simulink model "sampleModel7126_pp_1_1"  (R2018a)
settings: Solver=VariableStepAuto  StartTime=0.0  StopTime=10.0  RelTol=1e-3
undefined symbols (not defined in the file): DiscIntNeverNeededParam
libraries: simulink x367
(part 4 of 12)

== system sampleModel7126_pp_1_1/cfblk270 ==
  cfblk1 : Inport
  Action Port : ActionPort  ActionType=else
  cfblk11 : Subsystem  TreatAsAtomicUnit=on
  cfblk12 : Delay
  cfblk13 : Delay
  cfblk3 : UnitDelay  SampleTime=-1
  cfblk4 : Subsystem  TreatAsAtomicUnit=on
  cfblk5 : simulink/Continuous/PID Controller (2DOF)  Controller=PID  TimeDomain=Discrete-time  SampleTime=-1  IntegratorMethod=Forward Euler  FilterMethod=Forward Euler  Form=Parallel  UseFilter=on  ControllerParametersSource=internal  P=1  I=1  D=0  N=100  b=1  c=1  InitialConditionSource=internal  InitialConditionForIntegrator=0  InitialConditionForFilter=0  ExternalReset=none  LimitOutput=off  UpperSaturationLimit=inf  LowerSaturationLimit=-inf  LinearizeAsGain=off  AntiWindupMode=none  Kb=1  TrackingMode=off  Kt=1  PParamMin=[]  PParamMax=[]  IParamMin=[]  IParamMax=[]  DParamMin=[]  DParamMax=[]  NParamMin=[]  NParamMax=[]  bParamMin=[]  bParamMax=[]  cParamMin=[]  cParamMax=[]  KbParamMin=[]  KbParamMax=[]  KtParamMin=[]  KtParamMax=[]  POutMin=[]  POutMax=[]  IOutMin=[]  IOutMax=[]  DOutMin=[]  DOutMax=[]  NOutMin=[]  NOutMax=[]  bOutMin=[]  bOutMax=[]  cOutMin=[]  cOutMax=[]  KbOutMin=[]  KbOutMax=[]  KtOutMin=[]  KtOutMax=[]  IntegratorOutMin=[]  IntegratorOutMax=[]  FilterOutMin=[]  FilterOutMax=[]  SumOutMin=[]  SumOutMax=[]  Sum1OutMin=[]  Sum1OutMax=[]  Sum2OutMin=[]  Sum2OutMax=[]  Sum3OutMin=[]  Sum3OutMax=[]  SumI1OutMin=[]  SumI1OutMax=[]  SumI2OutMin=[]  SumI2OutMax=[]  SumI3OutMin=[]  SumI3OutMax=[]  SumDOutMin=[]  SumDOutMax=[]  SaturationOutMin=[]  SaturationOutMax=[]  IntegratorContinuousStateAttributes=''  IntegratorStateMustResolveToSignalObject=off  IntegratorRTWStateStorageClass=Auto  FilterContinuousStateAttributes=''  FilterStateMustResolveToSignalObject=off  FilterRTWStateStorageClass=Auto  DifferentiatorICPrevScaledInput=0  DifferentiatorOutMin=[]  DifferentiatorOutMax=[]  FilterDiffOutCoefMin=[]  FilterDiffOutCoefMax=[]  SumDenOutMin=[]  SumDenOutMax=[]  SumNumOutMin=[]  SumNumOutMax=[]  ReciprocalOutMin=[]  ReciprocalOutMax=[]  DivideOutMin=[]  DivideOutMax=[]  TunerSelectOption=Transfer Function Based (PID Tuner App)
  cfblk6 : simulink/Discrete/Transfer Fcn Lead or Lag  PoleZ=0.95  ZeroZ=0.75  ICPrevOutput=0.0  ICPrevInput=0.0  DoSatur=off
      settings: SourceProductName=Simulink  SourceProductBaseCode=SL
  cfblk7 : simulink/Continuous/PID Controller  Controller=PID  TimeDomain=Discrete-time  SampleTime=-1  IntegratorMethod=Forward Euler  FilterMethod=Forward Euler  Form=Parallel  UseFilter=on  ControllerParametersSource=internal  P=1  I=1  D=0  N=100  InitialConditionSource=internal  InitialConditionForIntegrator=0  InitialConditionForFilter=0  ExternalReset=none  LimitOutput=off  UpperSaturationLimit=inf  LowerSaturationLimit=-inf  LinearizeAsGain=off  AntiWindupMode=none  Kb=1  TrackingMode=off  Kt=1  PParamMin=[]  PParamMax=[]  IParamMin=[]  IParamMax=[]  DParamMin=[]  DParamMax=[]  NParamMin=[]  NParamMax=[]  KbParamMin=[]  KbParamMax=[]  KtParamMin=[]  KtParamMax=[]  POutMin=[]  POutMax=[]  IOutMin=[]  IOutMax=[]  DOutMin=[]  DOutMax=[]  NOutMin=[]  NOutMax=[]  KbOutMin=[]  KbOutMax=[]  KtOutMin=[]  KtOutMax=[]  IntegratorOutMin=[]  IntegratorOutMax=[]  FilterOutMin=[]  FilterOutMax=[]  SumOutMin=[]  SumOutMax=[]  SumI1OutMin=[]  SumI1OutMax=[]  SumI2OutMin=[]  SumI2OutMax=[]  SumI3OutMin=[]  SumI3OutMax=[]  SumDOutMin=[]  SumDOutMax=[]  SaturationOutMin=[]  SaturationOutMax=[]  IntegratorContinuousStateAttributes=''  IntegratorStateMustResolveToSignalObject=off  IntegratorRTWStateStorageClass=Auto  FilterContinuousStateAttributes=''  FilterStateMustResolveToSignalObject=off  FilterRTWStateStorageClass=Auto  DifferentiatorICPrevScaledInput=0  DifferentiatorOutMin=[]  DifferentiatorOutMax=[]  FilterDiffOutCoefMin=[]  FilterDiffOutCoefMax=[]  SumDenOutMin=[]  SumDenOutMax=[]  SumNumOutMin=[]  SumNumOutMax=[]  ReciprocalOutMin=[]  ReciprocalOutMax=[]  DivideOutMin=[]  DivideOutMax=[]  TunerSelectOption=Transfer Function Based (PID Tuner App)
  cfblk8 : Delay  ShowEnablePort=on
      settings: InputPortMap=u0,e6
  cfblk9 : Subsystem  TreatAsAtomicUnit=on
  cyemi_{675..687} (13 alike) : DataTypeConversion  OutDataTypeStr=double
  emi_2047 : Subsystem  TreatAsAtomicUnit=on
  emi_2049 : If  IfExpression=0 <= u1
  emi_2050 : DataTypeConversion  OutDataTypeStr=double
  emi_211 : Subsystem  TreatAsAtomicUnit=on
  emi_213 : If  IfExpression=0 <= u1  SampleTime=[1 0]
  emi_214 : DataTypeConversion  OutDataTypeStr=double
  emi_508 : Subsystem  TreatAsAtomicUnit=on
  emi_510 : If  IfExpression=0 <= u1  SampleTime=[1 0]
  emi_511 : DataTypeConversion  OutDataTypeStr=double
  cfblk2 : Outport
  cfblk10 : Outport  Port=2
  wires:
  cfblk5/1 -> cyemi_676/1, cyemi_679/1
  cfblk1/1 -> cfblk2/1, cfblk10/1, cyemi_683/1
  cfblk3/1 -> cyemi_681/1, cyemi_687/1, emi_511/1, emi_2050/1
  cyemi_676/1 -> cfblk12/1
  cyemi_677/1 -> cfblk13/1
  cfblk6/1 -> cyemi_677/1
  cyemi_678/1 -> cfblk3/1
  cfblk8/1 -> cyemi_678/1
  cyemi_680/1 -> cfblk5/1
  cyemi_681/1 -> cfblk5/2
  cyemi_682/1 -> cfblk6/1
  cyemi_683/1 -> cfblk7/1
  cyemi_684/1 -> cfblk8/1
  cfblk7/1 -> cyemi_684/1
  cyemi_685/1 -> cfblk8/2
  cfblk12/1 -> cyemi_685/1
  cfblk13/1 -> cyemi_686/1
  cyemi_679/1 -> cfblk4/1(emi_209)
  cfblk4/1(emi_210) -> cyemi_675/1
  emi_213/1 -> cfblk4/Action
  emi_213/2 -> emi_211/Action
  emi_214/1 -> emi_213/1
  cyemi_686/1 -> cfblk9/1(emi_505)
  cyemi_687/1 -> cfblk9/2(emi_506)
  cfblk9/1(emi_507) -> cyemi_682/1
  emi_510/1 -> cfblk9/Action
  emi_510/2 -> emi_508/Action
  emi_511/1 -> emi_510/1
  cyemi_675/1 -> cfblk11/1(emi_2045)
  cfblk11/1(emi_2046) -> emi_214/1, cyemi_680/1
  emi_2049/1 -> cfblk11/Action
  emi_2049/2 -> emi_2047/Action
  emi_2050/1 -> emi_2049/1

== system sampleModel7126_pp_1_1/cfblk271 ==
  cfblk1 : Inport
  cfblk14 : Inport  Port=2
  Action Port : ActionPort  ActionType=then
  cfblk10 : Subsystem  TreatAsAtomicUnit=on
  cfblk11 : simulink/Discrete/Difference  ICPrevInput=0.0  OutMin=[]  OutMax=[]  OutDataTypeStr=double  OutputDataTypeScalingMode=double  OutDataType=fixdt(1, 16)  OutScaling=2^-10  DoSatur=off
  cfblk12 : DiscreteZeroPole  Poles=[0 0.5]  Gain=1  SampleTime=-1
  cfblk13 : simulink/Continuous/PID Controller  Controller=PID  TimeDomain=Discrete-time  SampleTime=-1  IntegratorMethod=Forward Euler  FilterMethod=Forward Euler  Form=Parallel  UseFilter=on  ControllerParametersSource=internal  P=1  I=1  D=0  N=100  InitialConditionSource=internal  InitialConditionForIntegrator=0  InitialConditionForFilter=0  ExternalReset=none  LimitOutput=off  UpperSaturationLimit=inf  LowerSaturationLimit=-inf  LinearizeAsGain=off  AntiWindupMode=none  Kb=1  TrackingMode=off  Kt=1  PParamMin=[]  PParamMax=[]  IParamMin=[]  IParamMax=[]  DParamMin=[]  DParamMax=[]  NParamMin=[]  NParamMax=[]  KbParamMin=[]  KbParamMax=[]  KtParamMin=[]  KtParamMax=[]  POutMin=[]  POutMax=[]  IOutMin=[]  IOutMax=[]  DOutMin=[]  DOutMax=[]  NOutMin=[]  NOutMax=[]  KbOutMin=[]  KbOutMax=[]  KtOutMin=[]  KtOutMax=[]  IntegratorOutMin=[]  IntegratorOutMax=[]  FilterOutMin=[]  FilterOutMax=[]  SumOutMin=[]  SumOutMax=[]  SumI1OutMin=[]  SumI1OutMax=[]  SumI2OutMin=[]  SumI2OutMax=[]  SumI3OutMin=[]  SumI3OutMax=[]  SumDOutMin=[]  SumDOutMax=[]  SaturationOutMin=[]  SaturationOutMax=[]  IntegratorContinuousStateAttributes=''  IntegratorStateMustResolveToSignalObject=off  IntegratorRTWStateStorageClass=Auto  FilterContinuousStateAttributes=''  FilterStateMustResolveToSignalObject=off  FilterRTWStateStorageClass=Auto  DifferentiatorICPrevScaledInput=0  DifferentiatorOutMin=[]  DifferentiatorOutMax=[]  FilterDiffOutCoefMin=[]  FilterDiffOutCoefMax=[]  SumDenOutMin=[]  SumDenOutMax=[]  SumNumOutMin=[]  SumNumOutMax=[]  ReciprocalOutMin=[]  ReciprocalOutMax=[]  DivideOutMin=[]  DivideOutMax=[]  TunerSelectOption=Transfer Function Based (PID Tuner App)
  cfblk15 : Delay
  cfblk16 : Subsystem  TreatAsAtomicUnit=on
  cfblk3 : Subsystem  TreatAsAtomicUnit=on
  cfblk4 : Delay  DelayLengthSource=Input port
      settings: InputPortMap=u0,p1
  cfblk5 : simulink/Discrete/Difference  ICPrevInput=0.0  OutMin=[]  OutMax=[]  OutDataTypeStr=double  OutputDataTypeScalingMode=double  OutDataType=fixdt(1, 16)  OutScaling=2^-10  DoSatur=off
  cfblk6 : Delay  DelayLengthSource=Input port
      settings: InputPortMap=u0,p1
  cfblk7 : simulink/Continuous/PID Controller (2DOF)  Controller=PID  TimeDomain=Discrete-time  SampleTime=-1  IntegratorMethod=Forward Euler  FilterMethod=Forward Euler  Form=Parallel  UseFilter=on  ControllerParametersSource=internal  P=1  I=1  D=0  N=100  b=1  c=1  InitialConditionSource=internal  InitialConditionForIntegrator=0  InitialConditionForFilter=0  ExternalReset=none  LimitOutput=off  UpperSaturationLimit=inf  LowerSaturationLimit=-inf  LinearizeAsGain=off  AntiWindupMode=none  Kb=1  TrackingMode=off  Kt=1  PParamMin=[]  PParamMax=[]  IParamMin=[]  IParamMax=[]  DParamMin=[]  DParamMax=[]  NParamMin=[]  NParamMax=[]  bParamMin=[]  bParamMax=[]  cParamMin=[]  cParamMax=[]  KbParamMin=[]  KbParamMax=[]  KtParamMin=[]  KtParamMax=[]  POutMin=[]  POutMax=[]  IOutMin=[]  IOutMax=[]  DOutMin=[]  DOutMax=[]  NOutMin=[]  NOutMax=[]  bOutMin=[]  bOutMax=[]  cOutMin=[]  cOutMax=[]  KbOutMin=[]  KbOutMax=[]  KtOutMin=[]  KtOutMax=[]  IntegratorOutMin=[]  IntegratorOutMax=[]  FilterOutMin=[]  FilterOutMax=[]  SumOutMin=[]  SumOutMax=[]  Sum1OutMin=[]  Sum1OutMax=[]  Sum2OutMin=[]  Sum2OutMax=[]  Sum3OutMin=[]  Sum3OutMax=[]  SumI1OutMin=[]  SumI1OutMax=[]  SumI2OutMin=[]  SumI2OutMax=[]  SumI3OutMin=[]  SumI3OutMax=[]  SumDOutMin=[]  SumDOutMax=[]  SaturationOutMin=[]  SaturationOutMax=[]  IntegratorContinuousStateAttributes=''  IntegratorStateMustResolveToSignalObject=off  IntegratorRTWStateStorageClass=Auto  FilterContinuousStateAttributes=''  FilterStateMustResolveToSignalObject=off  FilterRTWStateStorageClass=Auto  DifferentiatorICPrevScaledInput=0  DifferentiatorOutMin=[]  DifferentiatorOutMax=[]  FilterDiffOutCoefMin=[]  FilterDiffOutCoefMax=[]  SumDenOutMin=[]  SumDenOutMax=[]  SumNumOutMin=[]  SumNumOutMax=[]  ReciprocalOutMin=[]  ReciprocalOutMax=[]  DivideOutMin=[]  DivideOutMax=[]  TunerSelectOption=Transfer Function Based (PID Tuner App)
  cfblk8 : UnitDelay  SampleTime=-1
  cfblk9 : simulink/Discrete/Transfer Fcn Real Zero  ZeroZ=0.75  ICPrevInput=0.0  DoSatur=off
      settings: SourceProductName=Simulink  SourceProductBaseCode=SL
  cyemi_{690..705} (16 alike) : DataTypeConversion  OutDataTypeStr=double
  emi_133 : Subsystem  TreatAsAtomicUnit=on
  emi_135 : If  IfExpression=Inf <= u1  SampleTime=[1 0]
  emi_136 : DataTypeConversion  OutDataTypeStr=double
  emi_1887 : Subsystem  TreatAsAtomicUnit=on
  emi_1889 : If  IfExpression=Inf <= u1
  emi_1890 : DataTypeConversion  OutDataTypeStr=double
  emi_1915 : Subsystem  TreatAsAtomicUnit=on
  emi_1917 : If  IfExpression=Inf <= u1  SampleTime=[1 0]
  emi_1918 : DataTypeConversion  OutDataTypeStr=double
  cfblk2 : Outport
  wires:
  cfblk13/1 -> cfblk2/1
  cfblk9/1 -> cyemi_690/1, cyemi_695/1
  cyemi_691/1 -> cfblk11/1
  cfblk14/1 -> cyemi_691/1
  cyemi_692/1 -> cfblk12/1
  cfblk1/1 -> cyemi_692/1
  cyemi_693/1 -> cfblk13/1
  cyemi_694/1 -> cfblk15/1
  cfblk5/1 -> cyemi_694/1
  cfblk6/1 -> cyemi_696/1
  cyemi_697/1 -> cfblk4/1
  cfblk8/1 -> cyemi_697/1
  cyemi_698/1 -> cfblk4/2
  cyemi_699/1 -> cfblk5/1
  cyemi_700/1 -> cfblk6/1
  cfblk15/1 -> cyemi_700/1, emi_1918/1
  cyemi_701/1 -> cfblk6/2
  cfblk12/1 -> cyemi_701/1, emi_136/1
  cyemi_702/1 -> cfblk7/1
  cfblk11/1 -> cyemi_702/1
  cyemi_703/1 -> cfblk7/2
  cyemi_704/1 -> cfblk8/1
  cfblk7/1 -> cyemi_704/1
  cyemi_705/1 -> cfblk9/1
  cfblk4/1 -> cyemi_705/1, emi_1890/1
  cyemi_695/1 -> cfblk16/1(emi_131)
  cfblk16/1(emi_132) -> cyemi_698/1
  emi_135/1 -> cfblk16/Action
  emi_135/2 -> emi_133/Action
  emi_136/1 -> emi_135/1
  cyemi_690/1 -> cfblk10/1(emi_1885)
  cfblk10/1(emi_1886) -> cyemi_699/1
  emi_1889/1 -> cfblk10/Action
  emi_1889/2 -> emi_1887/Action
  emi_1890/1 -> emi_1889/1
  cyemi_696/1 -> cfblk3/1(emi_1913)
  cfblk3/1(emi_1914) -> cyemi_703/1, cyemi_693/1
  emi_1917/1 -> cfblk3/Action
  emi_1917/2 -> emi_1915/Action
  emi_1918/1 -> emi_1917/1

== system sampleModel7126_pp_1_1/cfblk272 ==
  cfblk1 : Inport
  cfblk9 : Inport  Port=2
  Action Port : ActionPort  ActionType=else
  cfblk11 : Delay
  cfblk12 : Subsystem  TreatAsAtomicUnit=on
  cfblk13 : DataTypeConversion  OutDataTypeStr=double
  cfblk3 : Delay  ShowEnablePort=on
      settings: InputPortMap=u0,e6
  cfblk4 : Subsystem  TreatAsAtomicUnit=on
  cfblk5 : Subsystem  TreatAsAtomicUnit=on
  cfblk6 : Subsystem  TreatAsAtomicUnit=on
  cfblk7 : Subsystem  TreatAsAtomicUnit=on
  cfblk8 : UnitDelay  SampleTime=-1
  cyemi_{708..709,711..718} (10 alike) : DataTypeConversion  OutDataTypeStr=double
  cyemi_710 : DataTypeConversion  OutDataTypeStr=uint16
  emi_1033 : Subsystem  TreatAsAtomicUnit=on
  emi_{539,652,850,1035,1458} (5 alike) : If  IfExpression=0 <= u1  SampleTime=[1 0]
  emi_{540,653,851,1036,1459} (5 alike) : DataTypeConversion  OutDataTypeStr=double
  emi_1456 : Subsystem  TreatAsAtomicUnit=on
  emi_537 : Subsystem  TreatAsAtomicUnit=on
  emi_650 : Subsystem  TreatAsAtomicUnit=on
  emi_848 : Subsystem  TreatAsAtomicUnit=on
  cfblk2 : Outport
  cfblk10 : Outport  Port=2
  wires:
  cfblk3/1 -> cyemi_713/1, cyemi_718/1, emi_540/1, emi_1459/1
  cfblk1/1 -> cyemi_712/1, cyemi_715/1
  cyemi_708/1 -> cfblk11/1
  cyemi_710/1 -> cfblk13/1
  cfblk9/1 -> cyemi_710/1
  cyemi_711/1 -> cfblk3/1
  cfblk11/1 -> cyemi_711/1, emi_653/1
  cyemi_712/1 -> cfblk3/2
  cfblk8/1 -> cyemi_714/1
  cfblk13/1 -> cyemi_717/1, emi_1036/1
  cyemi_718/1 -> cfblk8/1
  cyemi_709/1 -> cfblk12/1(emi_535)
  cfblk12/1(emi_536) -> cyemi_716/1
  emi_539/1 -> cfblk12/Action
  emi_539/2 -> emi_537/Action
  emi_540/1 -> emi_539/1
  cyemi_714/1 -> cfblk5/1(emi_647)
  cyemi_715/1 -> cfblk5/2(emi_648)
  cfblk5/1(emi_649) -> cyemi_708/1
  emi_652/1 -> cfblk5/Action
  emi_652/2 -> emi_650/Action
  emi_653/1 -> emi_652/1
  cyemi_717/1 -> cfblk7/1(emi_846)
  cfblk7/1(emi_847) -> cyemi_709/1
  emi_850/1 -> cfblk7/Action
  emi_850/2 -> emi_848/Action
  emi_851/1 -> emi_850/1
  cyemi_713/1 -> cfblk4/1(emi_1031)
  cfblk4/1(emi_1032) -> emi_851/1, cfblk10/1
  emi_1035/1 -> cfblk4/Action
  emi_1035/2 -> emi_1033/Action
  emi_1036/1 -> emi_1035/1
  cyemi_716/1 -> cfblk6/1(emi_1454)
  cfblk6/1(emi_1455) -> cfblk2/1
  emi_1458/1 -> cfblk6/Action
  emi_1458/2 -> emi_1456/Action
  emi_1459/1 -> emi_1458/1

== system sampleModel7126_pp_1_1/cfblk273 ==
  cfblk1 : Inport
  cfblk8 : Inport  Port=2
  Action Port : ActionPort  ActionType=then
  cfblk10 : Subsystem  TreatAsAtomicUnit=on
  cfblk11 : Subsystem  TreatAsAtomicUnit=on
  cfblk12 : Delay
  cfblk3 : simulink/Discrete/Tapped Delay  vinit=0.0  samptime=-1  NumDelays=1  DelayOrder=Oldest  includeCurrent=off
  cfblk4 : UnitDelay  SampleTime=-1
  cfblk5 : DiscreteZeroPole  Poles=[0 0.5]  Gain=1  SampleTime=-1
  cfblk6 : Subsystem  TreatAsAtomicUnit=on
  cfblk7 : If  SampleTime=1
  cfblk9 : Subsystem  TreatAsAtomicUnit=on
  cyemi_{721..722,733..742} (12 alike) : DataTypeConversion  OutDataTypeStr=double
  emi_1994 : Subsystem  TreatAsAtomicUnit=on
  emi_1996 : If  IfExpression=-1.330790e+00 <= u1  SampleTime=[1 0]
  emi_1997 : DataTypeConversion  OutDataTypeStr=double
  emi_883 : Subsystem  TreatAsAtomicUnit=on
  emi_885 : If  IfExpression=-1.330790e+00 <= u1
  emi_886 : DataTypeConversion  OutDataTypeStr=double
  cfblk2 : Outport
  wires:
  cfblk3/1 -> cyemi_738/1, cyemi_742/1, emi_886/1, emi_1997/1
  cfblk9/1(cfblk2) -> cfblk2/1
  cfblk7/1 -> cfblk9/Action
  cfblk7/2 -> cfblk10/Action
  cyemi_721/1 -> cfblk10/1(cfblk1)
  cfblk4/1 -> cyemi_721/1
  cyemi_722/1 -> cfblk10/2(cfblk12)
  cfblk9/2(cfblk13) -> cyemi_733/1
  cyemi_734/1 -> cfblk12/1
  cfblk5/1 -> cyemi_734/1
  cyemi_735/1 -> cfblk3/1
  cfblk1/1 -> cyemi_735/1
  cyemi_736/1 -> cfblk4/1
  cfblk8/1 -> cyemi_736/1
  cyemi_737/1 -> cfblk5/1
  cfblk10/2(cfblk13) -> cyemi_737/1
  cyemi_739/1 -> cfblk7/1
  cyemi_740/1 -> cfblk9/1(cfblk1)
  cfblk10/1(cfblk2) -> cyemi_740/1
  cyemi_741/1 -> cfblk9/2(cfblk11)
  cfblk12/1 -> cyemi_741/1
  cyemi_742/1 -> cfblk9/3(cfblk12)
  cyemi_733/1 -> cfblk11/1(emi_881)
  cfblk11/1(emi_882) -> cyemi_739/1
  emi_885/1 -> cfblk11/Action
  emi_885/2 -> emi_883/Action
  emi_886/1 -> emi_885/1
  cyemi_738/1 -> cfblk6/1(emi_1992)
  cfblk6/1(emi_1993) -> cyemi_722/1
  emi_1996/1 -> cfblk6/Action
  emi_1996/2 -> emi_1994/Action
  emi_1997/1 -> emi_1996/1

== system sampleModel7126_pp_1_1/cfblk274 ==
  cfblk1 : Inport
  Action Port : ActionPort  ActionType=else
  cfblk10 : Delay
  cfblk3 : DiscreteTransferFcn
  cfblk4 : Subsystem  TreatAsAtomicUnit=on
  cfblk5 : Subsystem  TreatAsAtomicUnit=on
  cfblk6 : Subsystem  TreatAsAtomicUnit=on
  cfblk7 : Subsystem  TreatAsAtomicUnit=on
  cfblk9 : Delay
  cyemi_{754..762} (9 alike) : DataTypeConversion  OutDataTypeStr=double
  emi_1047 : Subsystem  TreatAsAtomicUnit=on
  emi_{397,893,1049,2099} (4 alike) : If  IfExpression=0 <= u1  SampleTime=[1 0]
  emi_{398,894,1050,2100} (4 alike) : DataTypeConversion  OutDataTypeStr=double
  emi_2097 : Subsystem  TreatAsAtomicUnit=on
  emi_395 : Subsystem  TreatAsAtomicUnit=on
  emi_891 : Subsystem  TreatAsAtomicUnit=on
  cfblk2 : Outport
  cfblk8 : Outport  Port=2
  wires:
  cfblk1/1 -> cfblk2/1
  cyemi_754/1 -> cfblk10/1
  cyemi_755/1 -> cfblk3/1
  cfblk10/1 -> cyemi_755/1
  cfblk9/1 -> cyemi_758/1, emi_894/1
  cfblk3/1 -> cyemi_759/1, emi_1050/1
  cyemi_762/1 -> cfblk9/1
  cyemi_756/1 -> cfblk4/1(emi_393)
  cfblk4/1(emi_394) -> cyemi_757/1
  emi_397/1 -> cfblk4/Action
  emi_397/2 -> emi_395/Action
  emi_398/1 -> emi_397/1
  cyemi_758/1 -> cfblk6/1(emi_888)
  cyemi_759/1 -> cfblk6/2(emi_889)
  cfblk6/1(emi_890) -> emi_398/1, cyemi_761/1, cyemi_760/1, emi_2100/1
  emi_893/1 -> cfblk6/Action
  emi_893/2 -> emi_891/Action
  emi_894/1 -> emi_893/1
  cyemi_757/1 -> cfblk5/1(emi_1045)
  cfblk5/1(emi_1046) -> cyemi_762/1, cyemi_754/1
  emi_1049/1 -> cfblk5/Action
  emi_1049/2 -> emi_1047/Action
  emi_1050/1 -> emi_1049/1
  cyemi_760/1 -> cfblk7/1(emi_2094)
  cyemi_761/1 -> cfblk7/2(emi_2095)
  cfblk7/1(emi_2096) -> cyemi_756/1, cfblk8/1
  emi_2099/1 -> cfblk7/Action
  emi_2099/2 -> emi_2097/Action
  emi_2100/1 -> emi_2099/1

== system sampleModel7126_pp_1_1/cfblk275 ==
  cfblk1 : Inport
  Action Port : ActionPort  ActionType=then
  cfblk10 : Subsystem  TreatAsAtomicUnit=on
  cfblk11 : Subsystem  TreatAsAtomicUnit=on
  cfblk12 : Delay
  cfblk13 : Delay
  cfblk3 : simulink/Discrete/Transfer Fcn Real Zero  ZeroZ=0.75  ICPrevInput=0.0  DoSatur=off
      settings: SourceProductName=Simulink  SourceProductBaseCode=SL
  cfblk4 : simulink/Discrete/Transfer Fcn Real Zero  ZeroZ=0.75  ICPrevInput=0.0  DoSatur=off
      settings: SourceProductName=Simulink  SourceProductBaseCode=SL
  cfblk5 : simulink/Continuous/PID Controller  Controller=PID  TimeDomain=Discrete-time  SampleTime=-1  IntegratorMethod=Forward Euler  FilterMethod=Forward Euler  Form=Parallel  UseFilter=on  ControllerParametersSource=internal  P=1  I=1  D=0  N=100  InitialConditionSource=internal  InitialConditionForIntegrator=0  InitialConditionForFilter=0  ExternalReset=none  LimitOutput=off  UpperSaturationLimit=inf  LowerSaturationLimit=-inf  LinearizeAsGain=off  AntiWindupMode=none  Kb=1  TrackingMode=off  Kt=1  PParamMin=[]  PParamMax=[]  IParamMin=[]  IParamMax=[]  DParamMin=[]  DParamMax=[]  NParamMin=[]  NParamMax=[]  KbParamMin=[]  KbParamMax=[]  KtParamMin=[]  KtParamMax=[]  POutMin=[]  POutMax=[]  IOutMin=[]  IOutMax=[]  DOutMin=[]  DOutMax=[]  NOutMin=[]  NOutMax=[]  KbOutMin=[]  KbOutMax=[]  KtOutMin=[]  KtOutMax=[]  IntegratorOutMin=[]  IntegratorOutMax=[]  FilterOutMin=[]  FilterOutMax=[]  SumOutMin=[]  SumOutMax=[]  SumI1OutMin=[]  SumI1OutMax=[]  SumI2OutMin=[]  SumI2OutMax=[]  SumI3OutMin=[]  SumI3OutMax=[]  SumDOutMin=[]  SumDOutMax=[]  SaturationOutMin=[]  SaturationOutMax=[]  IntegratorContinuousStateAttributes=''  IntegratorStateMustResolveToSignalObject=off  IntegratorRTWStateStorageClass=Auto  FilterContinuousStateAttributes=''  FilterStateMustResolveToSignalObject=off  FilterRTWStateStorageClass=Auto  DifferentiatorICPrevScaledInput=0  DifferentiatorOutMin=[]  DifferentiatorOutMax=[]  FilterDiffOutCoefMin=[]  FilterDiffOutCoefMax=[]  SumDenOutMin=[]  SumDenOutMax=[]  SumNumOutMin=[]  SumNumOutMax=[]  ReciprocalOutMin=[]  ReciprocalOutMax=[]  DivideOutMin=[]  DivideOutMax=[]  TunerSelectOption=Transfer Function Based (PID Tuner App)
  cfblk6 : simulink/Discrete/Difference  ICPrevInput=0.0  OutMin=[]  OutMax=[]  OutDataTypeStr=double  OutputDataTypeScalingMode=double  OutDataType=fixdt(1, 16)  OutScaling=2^-10  DoSatur=off
  cfblk7 : DiscreteStateSpace  SampleTime=-1
  cfblk8 : DiscreteIntegrator  SampleTime=-1  OutDataTypeStr=double  ICPrevOutput=DiscIntNeverNeededParam  ICPrevScaledInput=DiscIntNeverNeededParam
  cfblk9 : If  SampleTime=1
  cyemi_{764,777,792..800} (11 alike) : DataTypeConversion  OutDataTypeStr=double
  cfblk2 : Outport
  wires:
  cfblk1/1 -> cfblk2/1
  cfblk9/1 -> cfblk10/Action
  cfblk9/2 -> cfblk11/Action
  cyemi_764/1 -> cfblk10/1(cfblk1)
  cfblk11/2(cfblk15) -> cyemi_764/1
  cyemi_777/1 -> cfblk11/1(cfblk1)
  cfblk13/1 -> cyemi_777/1
  cyemi_792/1 -> cfblk12/1
  cfblk5/1 -> cyemi_792/1
  cyemi_793/1 -> cfblk13/1
  cfblk8/1 -> cyemi_793/1
  cyemi_794/1 -> cfblk3/1
  cfblk12/1 -> cyemi_794/1
  cyemi_795/1 -> cfblk4/1
  cfblk6/1 -> cyemi_795/1
  cyemi_796/1 -> cfblk5/1
  cfblk11/1(cfblk2) -> cyemi_796/1
  cyemi_797/1 -> cfblk6/1
  cfblk3/1 -> cyemi_797/1
  cyemi_798/1 -> cfblk7/1
  cfblk11/3(cfblk16) -> cyemi_798/1
  cyemi_799/1 -> cfblk8/1
  cfblk7/1 -> cyemi_799/1
  cyemi_800/1 -> cfblk9/1
  cfblk4/1 -> cyemi_800/1

== system sampleModel7126_pp_1_1/cfblk276 ==
  cfblk1 : Inport
  cfblk9 : Inport  Port=2
  cfblk10 : Inport  Port=3
  cfblk11 : Inport  Port=4
  Action Port : ActionPort  ActionType=else
  cfblk14 : Subsystem  TreatAsAtomicUnit=on
  cfblk3 : Subsystem  TreatAsAtomicUnit=on
  cfblk4 : Subsystem  TreatAsAtomicUnit=on
  cfblk5 : Subsystem  TreatAsAtomicUnit=on
  cfblk6 : Subsystem  TreatAsAtomicUnit=on
  cfblk7 : Subsystem  TreatAsAtomicUnit=on
  cfblk8 : Delay
  cyemi_{805..811} (7 alike) : DataTypeConversion  OutDataTypeStr=double
  cyemi_812 : DataTypeConversion  OutDataTypeStr=uint8
  emi_1105 : Subsystem  TreatAsAtomicUnit=on
  emi_{83,242,771,1107,1359} (5 alike) : If  IfExpression=0 <= u1  SampleTime=[1 0]
  emi_1108 : DataTypeConversion  OutDataTypeStr=double
  emi_1357 : Subsystem  TreatAsAtomicUnit=on
  emi_1360 : DataTypeConversion  OutDataTypeStr=uint8
  emi_1822 : Subsystem  TreatAsAtomicUnit=on
  emi_1824 : If  IfExpression=0 <= u1
  emi_1825 : DataTypeConversion  OutDataTypeStr=double
  emi_240 : Subsystem  TreatAsAtomicUnit=on
  emi_243 : DataTypeConversion  OutDataTypeStr=uint8
  emi_769 : Subsystem  TreatAsAtomicUnit=on
  emi_772 : DataTypeConversion  OutDataTypeStr=uint8
  emi_81 : Subsystem  TreatAsAtomicUnit=on
  emi_84 : DataTypeConversion  OutDataTypeStr=double
  cfblk2 : Outport
  cfblk12 : Outport  Port=2
  cfblk13 : Outport  Port=3
  wires:
  cfblk9/1 -> cfblk2/1
  cfblk11/1 -> cfblk13/1
  cfblk8/1 -> cfblk12/1, emi_243/1, emi_772/1, emi_1360/1
  cfblk10/1 -> cyemi_809/1
  cyemi_812/1 -> cfblk8/1
  cfblk1/1 -> cyemi_812/1
  cyemi_807/1 -> cfblk4/1(emi_79)
  cfblk4/1(emi_80) -> cyemi_811/1, emi_1825/1
  emi_83/1 -> cfblk4/Action
  emi_83/2 -> emi_81/Action
  emi_84/1 -> emi_83/1
  cyemi_806/1 -> cfblk3/1(emi_238)
  cfblk3/1(emi_239) -> cyemi_808/1
  emi_242/1 -> cfblk3/Action
  emi_242/2 -> emi_240/Action
  emi_243/1 -> emi_242/1
  cyemi_808/1 -> cfblk5/1(emi_767)
  cfblk5/1(emi_768) -> cyemi_807/1
  emi_771/1 -> cfblk5/Action
  emi_771/2 -> emi_769/Action
  emi_772/1 -> emi_771/1
  cyemi_809/1 -> cfblk6/1(emi_1102)
  cyemi_810/1 -> cfblk6/2(emi_1103)
  cfblk6/1(emi_1104) -> cyemi_805/1
  emi_1107/1 -> cfblk6/Action
  emi_1107/2 -> emi_1105/Action
  emi_1108/1 -> emi_1107/1
  cyemi_811/1 -> cfblk7/1(emi_1355)
  cfblk7/1(emi_1356) -> cyemi_810/1
  emi_1359/1 -> cfblk7/Action
  emi_1359/2 -> emi_1357/Action
  emi_1360/1 -> emi_1359/1
  cyemi_805/1 -> cfblk14/1(emi_1820)
  cfblk14/1(emi_1821) -> emi_1108/1, emi_84/1, cyemi_806/1
  emi_1824/1 -> cfblk14/Action
  emi_1824/2 -> emi_1822/Action
  emi_1825/1 -> emi_1824/1

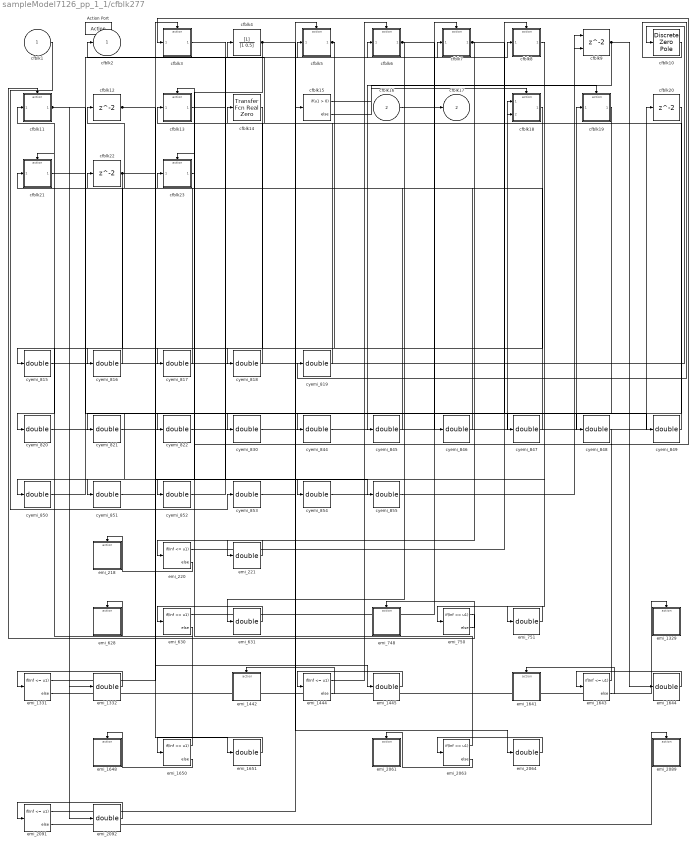
== system sampleModel7126_pp_1_1/cfblk277 ==
  cfblk1 : Inport
  cfblk16 : Inport  Port=2
  Action Port : ActionPort  ActionType=then
  cfblk10 : DiscreteZeroPole  Poles=[0 0.5]  Gain=1  SampleTime=-1
  cfblk11 : Subsystem  TreatAsAtomicUnit=on
  cfblk12 : Delay
  cfblk13 : Subsystem  TreatAsAtomicUnit=on
  cfblk14 : simulink/Discrete/Transfer Fcn Real Zero  ZeroZ=0.75  ICPrevInput=0.0  DoSatur=off
      settings: SourceProductName=Simulink  SourceProductBaseCode=SL
  cfblk15 : If  SampleTime=1
  cfblk18 : Subsystem  TreatAsAtomicUnit=on
  cfblk19 : Subsystem  TreatAsAtomicUnit=on
  cfblk20 : Delay
  cfblk21 : Subsystem  TreatAsAtomicUnit=on
  cfblk22 : Delay
  cfblk23 : Subsystem  TreatAsAtomicUnit=on
  cfblk3 : Subsystem  TreatAsAtomicUnit=on
  cfblk4 : DiscreteFilter
  cfblk5 : Subsystem  TreatAsAtomicUnit=on
  cfblk6 : Subsystem  TreatAsAtomicUnit=on
  cfblk7 : Subsystem  TreatAsAtomicUnit=on
  cfblk8 : Subsystem  TreatAsAtomicUnit=on
  cfblk9 : Delay  ShowEnablePort=on
      settings: InputPortMap=u0,e6
  cyemi_{815..822,830,844..855} (21 alike) : DataTypeConversion  OutDataTypeStr=double
  emi_1329 : Subsystem  TreatAsAtomicUnit=on
  emi_{220,630,750,1331,1643,1650,2063,2091} (8 alike) : If  IfExpression=Inf <= u1  SampleTime=[1 0]
  emi_{221,631,751,1332,1445,1644,1651,2064,2092} (9 alike) : DataTypeConversion  OutDataTypeStr=double
  emi_1442 : Subsystem  TreatAsAtomicUnit=on
  emi_1444 : If  IfExpression=Inf <= u1  SampleTime=[0 1]
  emi_1641 : Subsystem  TreatAsAtomicUnit=on
  emi_1648 : Subsystem  TreatAsAtomicUnit=on
  emi_2061 : Subsystem  TreatAsAtomicUnit=on
  emi_2089 : Subsystem  TreatAsAtomicUnit=on
  emi_218 : Subsystem  TreatAsAtomicUnit=on
  emi_628 : Subsystem  TreatAsAtomicUnit=on
  emi_748 : Subsystem  TreatAsAtomicUnit=on
  cfblk2 : Outport
  cfblk17 : Outport  Port=2
  wires:
  cfblk12/1 -> cyemi_830/1, cyemi_855/1, emi_1445/1
  cfblk16/1 -> cfblk17/1
  cfblk4/1 -> cfblk2/1, cyemi_822/1, emi_2064/1
  cfblk15/1 -> cfblk18/Action
  cfblk15/2 -> cfblk19/Action
  cyemi_815/1 -> cfblk10/1
  cfblk18/1(cfblk2) -> cyemi_816/1
  cyemi_817/1 -> cfblk12/1
  cfblk14/1 -> cyemi_818/1
  cyemi_819/1 -> cfblk14/1
  cfblk10/1 -> cyemi_819/1
  cyemi_820/1 -> cfblk15/1
  cfblk22/1 -> cyemi_820/1, emi_1651/1
  cyemi_821/1 -> cfblk18/1(cfblk1)
  cfblk20/1 -> cyemi_821/1
  cyemi_822/1 -> cfblk18/2(cfblk8)
  cyemi_830/1 -> cfblk19/1(cfblk1)
  cyemi_844/1 -> cfblk20/1
  cfblk9/1 -> cyemi_845/1, emi_751/1, emi_1644/1
  cyemi_846/1 -> cfblk22/1
  cyemi_849/1 -> cfblk4/1
  cfblk19/1(cfblk2) -> cyemi_851/1
  cfblk1/1 -> cyemi_853/1
  cyemi_854/1 -> cfblk9/1
  cyemi_855/1 -> cfblk9/2
  cyemi_853/1 -> cfblk8/1(emi_216)
  cfblk8/1(emi_217) -> cyemi_852/1
  emi_220/1 -> cfblk8/Action
  emi_220/2 -> emi_218/Action
  emi_221/1 -> emi_220/1
  cyemi_852/1 -> cfblk7/1(emi_626)
  cfblk7/1(emi_627) -> emi_221/1, cyemi_849/1
  emi_630/1 -> cfblk7/Action
  emi_630/2 -> emi_628/Action
  emi_631/1 -> emi_630/1
  cyemi_816/1 -> cfblk11/1(emi_746)
  cfblk11/1(emi_747) -> cyemi_844/1, emi_1332/1, emi_2092/1
  emi_750/1 -> cfblk11/Action
  emi_750/2 -> emi_748/Action
  emi_751/1 -> emi_750/1
  cyemi_848/1 -> cfblk3/1(emi_1327)
  cfblk3/1(emi_1328) -> cyemi_854/1
  emi_1331/1 -> cfblk3/Action
  emi_1331/2 -> emi_1329/Action
  emi_1332/1 -> emi_1331/1
  cyemi_851/1 -> cfblk6/1(emi_1440)
  cfblk6/1(emi_1441) -> emi_631/1, cyemi_846/1
  emi_1444/1 -> cfblk6/Action
  emi_1444/2 -> emi_1442/Action
  emi_1445/1 -> emi_1444/1
  cyemi_818/1 -> cfblk13/1(emi_1639)
  cfblk13/1(emi_1640) -> cyemi_847/1
  emi_1643/1 -> cfblk13/Action
  emi_1643/2 -> emi_1641/Action
  emi_1644/1 -> emi_1643/1
  cyemi_845/1 -> cfblk21/1(emi_1646)
  cfblk21/1(emi_1647) -> cyemi_848/1
  emi_1650/1 -> cfblk21/Action
  emi_1650/2 -> emi_1648/Action
  emi_1651/1 -> emi_1650/1
  cyemi_847/1 -> cfblk23/1(emi_2059)
  cfblk23/1(emi_2060) -> cyemi_850/1
  emi_2063/1 -> cfblk23/Action
  emi_2063/2 -> emi_2061/Action
  emi_2064/1 -> emi_2063/1
  cyemi_850/1 -> cfblk5/1(emi_2087)
  cfblk5/1(emi_2088) -> cyemi_817/1, cyemi_815/1
  emi_2091/1 -> cfblk5/Action
  emi_2091/2 -> emi_2089/Action
  emi_2092/1 -> emi_2091/1

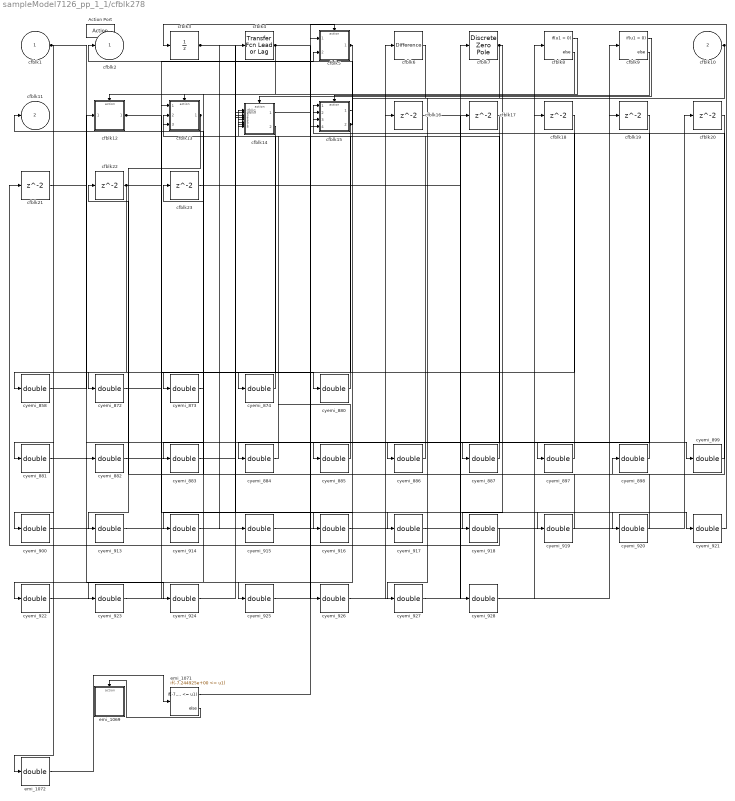
== system sampleModel7126_pp_1_1/cfblk278 ==
  cfblk1 : Inport
  cfblk10 : Inport  Port=2
  Action Port : ActionPort  ActionType=else
  cfblk12 : Subsystem  TreatAsAtomicUnit=on
  cfblk13 : Subsystem  TreatAsAtomicUnit=on
  cfblk14 : Subsystem  TreatAsAtomicUnit=on
  cfblk15 : Subsystem  TreatAsAtomicUnit=on
  cfblk{16..23} (8 alike) : Delay
  cfblk3 : UnitDelay  SampleTime=-1
  cfblk4 : simulink/Discrete/Transfer Fcn Lead or Lag  PoleZ=0.95  ZeroZ=0.75  ICPrevOutput=0.0  ICPrevInput=0.0  DoSatur=off
      settings: SourceProductName=Simulink  SourceProductBaseCode=SL
  cfblk5 : Subsystem  TreatAsAtomicUnit=on
  cfblk6 : simulink/Discrete/Difference  ICPrevInput=0.0  OutMin=[]  OutMax=[]  OutDataTypeStr=double  OutputDataTypeScalingMode=double  OutDataType=fixdt(1, 16)  OutScaling=2^-10  DoSatur=off
  cfblk7 : DiscreteZeroPole  Poles=[0 0.5]  Gain=1  SampleTime=-1
  cfblk8 : If  SampleTime=1
  cfblk9 : If  SampleTime=1
  cyemi_{858,872..874,880..887,897..900,913..928} (32 alike) : DataTypeConversion  OutDataTypeStr=double
  emi_1069 : Subsystem  TreatAsAtomicUnit=on
  emi_1071 : If  IfExpression=-7.244925e+00 <= u1  SampleTime=[1 0]
  emi_1072 : DataTypeConversion  OutDataTypeStr=double
  cfblk2 : Outport
  cfblk11 : Outport  Port=2
  wires:
  cfblk13/1(cfblk2) -> cfblk11/1, cyemi_913/1
  cfblk12/1(cfblk2) -> cyemi_917/1, cyemi_921/1
  cfblk1/1 -> cyemi_881/1, cyemi_897/1, cyemi_900/1, cyemi_924/1
  cfblk7/1 -> cyemi_918/1, cyemi_927/1
  cfblk4/1 -> cyemi_919/1, cyemi_920/1, cyemi_923/1
  cfblk3/1 -> cyemi_915/1, cyemi_916/1
  cfblk10/1 -> cyemi_886/1, cyemi_925/1
  cfblk15/2(cfblk16) -> cfblk2/1, cyemi_883/1, cyemi_885/1
  cfblk8/1 -> cfblk12/Action
  cfblk8/2 -> cfblk13/Action
  cfblk9/1 -> cfblk14/Action
  cfblk9/2 -> cfblk15/Action
  cyemi_858/1 -> cfblk12/1(cfblk1)
  cfblk14/2(cfblk16) -> cyemi_858/1
  cyemi_872/1 -> cfblk13/1(cfblk1)
  cyemi_873/1 -> cfblk13/2(cfblk8)
  cfblk6/1 -> cyemi_873/1
  cyemi_874/1 -> cfblk13/3(cfblk9)
  cfblk18/1 -> cyemi_874/1
  cyemi_880/1 -> cfblk14/1(cfblk1)
  cfblk22/1 -> cyemi_880/1, emi_1072/1
  cyemi_881/1 -> cfblk14/2(cfblk9)
  cyemi_882/1 -> cfblk14/3(cfblk10)
  cfblk21/1 -> cyemi_882/1
  cyemi_883/1 -> cfblk14/4(cfblk11)
  cyemi_884/1 -> cfblk14/5(cfblk12)
  cfblk17/1 -> cyemi_884/1
  cyemi_885/1 -> cfblk14/6(cfblk13)
  cyemi_886/1 -> cfblk14/7(cfblk14)
  cyemi_887/1 -> cfblk14/8(cfblk15)
  cfblk19/1 -> cyemi_887/1
  cyemi_897/1 -> cfblk15/1(cfblk1)
  cyemi_898/1 -> cfblk15/2(cfblk13)
  cfblk20/1 -> cyemi_898/1
  cyemi_899/1 -> cfblk15/3(cfblk14)
  cfblk16/1 -> cyemi_899/1
  cyemi_900/1 -> cfblk15/4(cfblk15)
  cyemi_913/1 -> cfblk16/1
  cyemi_914/1 -> cfblk17/1
  cyemi_915/1 -> cfblk18/1
  cyemi_916/1 -> cfblk19/1
  cyemi_917/1 -> cfblk20/1
  cyemi_918/1 -> cfblk21/1
  cyemi_919/1 -> cfblk22/1
  cyemi_920/1 -> cfblk23/1
  cyemi_921/1 -> cfblk3/1
  cyemi_922/1 -> cfblk4/1
  cfblk15/1(cfblk2) -> cyemi_922/1
  cyemi_925/1 -> cfblk6/1
  cyemi_926/1 -> cfblk7/1
  cfblk14/1(cfblk2) -> cyemi_926/1
  cyemi_927/1 -> cfblk8/1
  cyemi_928/1 -> cfblk9/1
  cfblk23/1 -> cyemi_928/1
  cyemi_923/1 -> cfblk5/1(emi_1066)
  cyemi_924/1 -> cfblk5/2(emi_1067)
  cfblk5/1(emi_1068) -> cyemi_914/1, cyemi_872/1
  emi_1071/1 -> cfblk5/Action
  emi_1071/2 -> emi_1069/Action
  emi_1072/1 -> emi_1071/1

== system sampleModel7126_pp_1_1/cfblk279 ==
  cfblk1 : Inport
  cfblk8 : Inport  Port=2
  Action Port : ActionPort  ActionType=then
  cfblk10 : Subsystem  TreatAsAtomicUnit=on
  cfblk11 : Subsystem  TreatAsAtomicUnit=on
  cfblk3 : Subsystem  TreatAsAtomicUnit=on
  cfblk4 : Subsystem  TreatAsAtomicUnit=on
  cfblk5 : DiscreteTransferFcn
  cfblk6 : DiscreteStateSpace  SampleTime=-1
  cfblk7 : Subsystem  TreatAsAtomicUnit=on
  cyemi_{931..938} (8 alike) : DataTypeConversion  OutDataTypeStr=double
  emi_1090 : Subsystem  TreatAsAtomicUnit=on
  emi_1092 : If  IfExpression=0 <= u1
  emi_{6,688,809,1093,1178} (5 alike) : DataTypeConversion  OutDataTypeStr=double
  emi_1175 : Subsystem  TreatAsAtomicUnit=on
  emi_{5,687,808,1177} (4 alike) : If  IfExpression=0 <= u1  SampleTime=[1 0]
  emi_3 : Subsystem  TreatAsAtomicUnit=on
  emi_685 : Subsystem  TreatAsAtomicUnit=on
  emi_806 : Subsystem  TreatAsAtomicUnit=on
  cfblk2 : Outport
  cfblk9 : Outport  Port=2
  wires:
  cfblk1/1 -> cfblk9/1
  cfblk5/1 -> cfblk2/1, cyemi_931/1, emi_1093/1
  cfblk6/1 -> cyemi_932/1, emi_6/1, emi_688/1
  cfblk8/1 -> cyemi_933/1
  cyemi_935/1 -> cfblk5/1
  cyemi_936/1 -> cfblk6/1
  cyemi_934/1 -> cfblk4/1(emi_1)
  cfblk4/1(emi_2) -> cyemi_936/1
  emi_5/1 -> cfblk4/Action
  emi_5/2 -> emi_3/Action
  emi_6/1 -> emi_5/1
  cyemi_932/1 -> cfblk11/1(emi_683)
  cfblk11/1(emi_684) -> cyemi_934/1, emi_809/1, emi_1178/1
  emi_687/1 -> cfblk11/Action
  emi_687/2 -> emi_685/Action
  emi_688/1 -> emi_687/1
  cyemi_937/1 -> cfblk7/1(emi_803)
  cyemi_938/1 -> cfblk7/2(emi_804)
  cfblk7/1(emi_805) -> cyemi_935/1
  emi_808/1 -> cfblk7/Action
  emi_808/2 -> emi_806/Action
  emi_809/1 -> emi_808/1
  cyemi_931/1 -> cfblk10/1(emi_1088)
  cfblk10/1(emi_1089) -> cyemi_938/1
  emi_1092/1 -> cfblk10/Action
  emi_1092/2 -> emi_1090/Action
  emi_1093/1 -> emi_1092/1
  cyemi_933/1 -> cfblk3/1(emi_1173)
  cfblk3/1(emi_1174) -> cyemi_937/1
  emi_1177/1 -> cfblk3/Action
  emi_1177/2 -> emi_1175/Action
  emi_1178/1 -> emi_1177/1

== system sampleModel7126_pp_1_1/cfblk280 ==
  cfblk1 : Inport
  cfblk10 : Inport  Port=2
  Action Port : ActionPort  ActionType=else
  cfblk13 : Subsystem  TreatAsAtomicUnit=on
  cfblk14 : Subsystem  TreatAsAtomicUnit=on
  cfblk15 : Delay
  cfblk16 : Subsystem  TreatAsAtomicUnit=on
  cfblk3 : Delay  DelayLengthSource=Input port
      settings: InputPortMap=u0,p1
  cfblk4 : Subsystem  TreatAsAtomicUnit=on
  cfblk5 : simulink/Discrete/Transfer Fcn First Order  PoleZ=0.95  ICPrevOutput=0.0  DoSatur=off
      settings: SourceProductName=Simulink
  cfblk6 : simulink/Discrete/Tapped Delay  vinit=0.0  samptime=-1  NumDelays=1  DelayOrder=Oldest  includeCurrent=off
  cfblk7 : simulink/Discrete/Transfer Fcn Lead or Lag  PoleZ=0.95  ZeroZ=0.75  ICPrevOutput=0.0  ICPrevInput=0.0  DoSatur=off
      settings: SourceProductName=Simulink  SourceProductBaseCode=SL
  cfblk8 : Delay  ShowEnablePort=on
      settings: InputPortMap=u0,e6
  cfblk9 : If  SampleTime=1
  cyemi_{942,961,963,965,969..970} (6 alike) : DataTypeConversion  OutDataTypeStr=double
  cyemi_{951,953,966..968} (5 alike) : DataTypeConversion  OutDataTypeStr=uint8
  cyemi_952 : DataTypeConversion  OutDataTypeStr=fixdt('ufix8_E6')
  cyemi_960 : DataTypeConversion  OutDataTypeStr=fixdt('ufix8_E6')
  cyemi_962 : DataTypeConversion  OutDataTypeStr=fixdt('ufix8_E3')
  cyemi_964 : DataTypeConversion  OutDataTypeStr=fixdt('ufix8_E3')
  emi_310 : Subsystem  TreatAsAtomicUnit=on
  emi_312 : If  IfExpression=Inf <= u1  SampleTime=[1 0]
  emi_313 : DataTypeConversion  OutDataTypeStr=double
  emi_360 : Subsystem  TreatAsAtomicUnit=on
  emi_362 : If  IfExpression=Inf <= u1  SampleTime=[1 0]
  emi_363 : DataTypeConversion  OutDataTypeStr=double
  cfblk2 : Outport
  cfblk11 : Outport  Port=2
  cfblk12 : Outport  Port=3
  wires:
  cfblk1/1 -> cfblk11/1, cyemi_953/1, cyemi_966/1
  cfblk10/1 -> cyemi_942/1, cyemi_969/1
  cfblk7/1 -> cfblk12/1, cyemi_962/1
  cfblk14/2(cfblk10) -> cfblk2/1
  cfblk9/1 -> cfblk13/Action
  cfblk9/2 -> cfblk14/Action
  cyemi_942/1 -> cfblk13/1(cfblk1)
  cyemi_951/1 -> cfblk14/1(cfblk1)
  cfblk6/1 -> cyemi_951/1
  cyemi_952/1 -> cfblk14/2(cfblk8)
  cfblk15/1 -> cyemi_952/1
  cyemi_953/1 -> cfblk14/3(cfblk9)
  cyemi_960/1 -> cfblk15/1
  cfblk13/2(cfblk8) -> cyemi_961/1
  cyemi_962/1 -> cfblk3/1
  cyemi_963/1 -> cfblk3/2
  cfblk5/1 -> cyemi_963/1
  cfblk3/1 -> cyemi_964/1
  cyemi_965/1 -> cfblk5/1
  cfblk13/1(cfblk2) -> cyemi_965/1
  cyemi_966/1 -> cfblk6/1
  cyemi_967/1 -> cfblk7/1
  cfblk8/1 -> cyemi_967/1, emi_313/1
  cyemi_968/1 -> cfblk8/1
  cfblk14/1(cfblk2) -> cyemi_968/1
  cyemi_969/1 -> cfblk8/2
  cyemi_970/1 -> cfblk9/1
  cyemi_961/1 -> cfblk16/1(emi_308)
  cfblk16/1(emi_309) -> cyemi_970/1, emi_363/1
  emi_312/1 -> cfblk16/Action
  emi_312/2 -> emi_310/Action
  emi_313/1 -> emi_312/1
  cyemi_964/1 -> cfblk4/1(emi_358)
  cfblk4/1(emi_359) -> cyemi_960/1
  emi_362/1 -> cfblk4/Action
  emi_362/2 -> emi_360/Action
  emi_363/1 -> emi_362/1

== system sampleModel7126_pp_1_1/cfblk281 ==
  cfblk1 : Inport
  cfblk12 : Inport  Port=2
  cfblk13 : Inport  Port=3
  Action Port : ActionPort  ActionType=then
  cfblk10 : Delay
  cfblk11 : simulink/Discrete/Transfer Fcn First Order  PoleZ=0.95  ICPrevOutput=0.0  DoSatur=off
      settings: SourceProductName=Simulink
  cfblk3 : Subsystem  TreatAsAtomicUnit=on
  cfblk4 : simulink/Continuous/PID Controller  Controller=PID  TimeDomain=Discrete-time  SampleTime=-1  IntegratorMethod=Forward Euler  FilterMethod=Forward Euler  Form=Parallel  UseFilter=on  ControllerParametersSource=internal  P=1  I=1  D=0  N=100  InitialConditionSource=internal  InitialConditionForIntegrator=0  InitialConditionForFilter=0  ExternalReset=none  LimitOutput=off  UpperSaturationLimit=inf  LowerSaturationLimit=-inf  LinearizeAsGain=off  AntiWindupMode=none  Kb=1  TrackingMode=off  Kt=1  PParamMin=[]  PParamMax=[]  IParamMin=[]  IParamMax=[]  DParamMin=[]  DParamMax=[]  NParamMin=[]  NParamMax=[]  KbParamMin=[]  KbParamMax=[]  KtParamMin=[]  KtParamMax=[]  POutMin=[]  POutMax=[]  IOutMin=[]  IOutMax=[]  DOutMin=[]  DOutMax=[]  NOutMin=[]  NOutMax=[]  KbOutMin=[]  KbOutMax=[]  KtOutMin=[]  KtOutMax=[]  IntegratorOutMin=[]  IntegratorOutMax=[]  FilterOutMin=[]  FilterOutMax=[]  SumOutMin=[]  SumOutMax=[]  SumI1OutMin=[]  SumI1OutMax=[]  SumI2OutMin=[]  SumI2OutMax=[]  SumI3OutMin=[]  SumI3OutMax=[]  SumDOutMin=[]  SumDOutMax=[]  SaturationOutMin=[]  SaturationOutMax=[]  IntegratorContinuousStateAttributes=''  IntegratorStateMustResolveToSignalObject=off  IntegratorRTWStateStorageClass=Auto  FilterContinuousStateAttributes=''  FilterStateMustResolveToSignalObject=off  FilterRTWStateStorageClass=Auto  DifferentiatorICPrevScaledInput=0  DifferentiatorOutMin=[]  DifferentiatorOutMax=[]  FilterDiffOutCoefMin=[]  FilterDiffOutCoefMax=[]  SumDenOutMin=[]  SumDenOutMax=[]  SumNumOutMin=[]  SumNumOutMax=[]  ReciprocalOutMin=[]  ReciprocalOutMax=[]  DivideOutMin=[]  DivideOutMax=[]  TunerSelectOption=Transfer Function Based (PID Tuner App)
  cfblk5 : Delay  ShowEnablePort=on
      settings: InputPortMap=u0,e6
  cfblk6 : Delay
  cfblk7 : Delay  DelayLengthSource=Input port
      settings: InputPortMap=u0,p1
  cfblk8 : DiscreteStateSpace  SampleTime=-1
  cfblk9 : DiscreteFilter
  cyemi_{974..984} (11 alike) : DataTypeConversion  OutDataTypeStr=double
  emi_140 : Subsystem  TreatAsAtomicUnit=on
  emi_142 : If  IfExpression=0 <= u1  SampleTime=[1 0]
  emi_143 : DataTypeConversion  OutDataTypeStr=double
  cfblk2 : Outport
  wires:
  cfblk7/1 -> cfblk2/1
  cyemi_974/1 -> cfblk10/1
  cfblk5/1 -> cyemi_974/1
  cyemi_975/1 -> cfblk11/1
  cfblk8/1 -> cyemi_975/1, emi_143/1
  cfblk4/1 -> cyemi_976/1
  cyemi_977/1 -> cfblk4/1
  cfblk6/1 -> cyemi_977/1
  cyemi_978/1 -> cfblk5/1
  cfblk9/1 -> cyemi_978/1
  cyemi_979/1 -> cfblk5/2
  cfblk11/1 -> cyemi_979/1
  cyemi_980/1 -> cfblk6/1
  cfblk1/1 -> cyemi_980/1
  cyemi_981/1 -> cfblk7/1
  cfblk12/1 -> cyemi_981/1
  cyemi_982/1 -> cfblk7/2
  cfblk10/1 -> cyemi_982/1
  cyemi_983/1 -> cfblk8/1
  cfblk13/1 -> cyemi_983/1
  cyemi_984/1 -> cfblk9/1
  cyemi_976/1 -> cfblk3/1(emi_138)
  cfblk3/1(emi_139) -> cyemi_984/1
  emi_142/1 -> cfblk3/Action
  emi_142/2 -> emi_140/Action
  emi_143/1 -> emi_142/1

== system sampleModel7126_pp_1_1/cfblk282 ==
  cfblk1 : Inport
  cfblk10 : Inport  Port=2
  cfblk11 : Inport  Port=3
  Action Port : ActionPort  ActionType=else
  cfblk16 : Delay
  cfblk17 : Delay
  cfblk3 : Subsystem  TreatAsAtomicUnit=on
  cfblk4 : Subsystem  TreatAsAtomicUnit=on
  cfblk5 : Subsystem  TreatAsAtomicUnit=on
  cfblk6 : simulink/Discrete/Tapped Delay  vinit=0.0  samptime=-1  NumDelays=1  DelayOrder=Oldest  includeCurrent=off
  cfblk7 : Subsystem  TreatAsAtomicUnit=on
  cfblk8 : Delay  DelayLengthSource=Input port
      settings: InputPortMap=u0,p1
  cfblk9 : DiscreteFir
  cyemi_{988..998} (11 alike) : DataTypeConversion  OutDataTypeStr=double
  emi_1019 : Subsystem  TreatAsAtomicUnit=on
  emi_{1021,1529,1852,1925} (4 alike) : If  IfExpression=0 <= u1  SampleTime=[1 0]
  emi_{1022,1530,1853,1926} (4 alike) : DataTypeConversion  OutDataTypeStr=double
  emi_1527 : Subsystem  TreatAsAtomicUnit=on
  emi_1850 : Subsystem  TreatAsAtomicUnit=on
  emi_1923 : Subsystem  TreatAsAtomicUnit=on
  cfblk2 : Outport
  cfblk12 : Outport  Port=2
  cfblk13 : Outport  Port=3
  cfblk14 : Outport  Port=4
  cfblk15 : Outport  Port=5
  wires:
  cfblk8/1 -> cfblk15/1, cfblk12/1, cyemi_991/1, cyemi_995/1
  cfblk11/1 -> cfblk2/1, cfblk13/1
  cyemi_988/1 -> cfblk16/1
  cyemi_989/1 -> cfblk17/1
  cfblk9/1 -> cyemi_989/1, emi_1022/1, emi_1926/1
  cfblk16/1 -> cyemi_992/1
  cfblk1/1 -> cyemi_993/1
  cyemi_994/1 -> cfblk6/1
  cfblk17/1 -> cyemi_994/1
  cyemi_996/1 -> cfblk8/1
  cyemi_997/1 -> cfblk8/2
  cfblk10/1 -> cyemi_997/1
  cyemi_998/1 -> cfblk9/1
  cfblk6/1 -> cyemi_998/1, emi_1530/1
  cyemi_991/1 -> cfblk4/1(emi_1017)
  cfblk4/1(emi_1018) -> cfblk14/1
  emi_1021/1 -> cfblk4/Action
  emi_1021/2 -> emi_1019/Action
  emi_1022/1 -> emi_1021/1
  cyemi_995/1 -> cfblk7/1(emi_1525)
  cfblk7/1(emi_1526) -> cyemi_988/1
  emi_1529/1 -> cfblk7/Action
  emi_1529/2 -> emi_1527/Action
  emi_1530/1 -> emi_1529/1
  cyemi_990/1 -> cfblk3/1(emi_1848)
  cfblk3/1(emi_1849) -> cyemi_996/1
  emi_1852/1 -> cfblk3/Action
  emi_1852/2 -> emi_1850/Action
  emi_1853/1 -> emi_1852/1
  cyemi_992/1 -> cfblk5/1(emi_1920)
  cyemi_993/1 -> cfblk5/2(emi_1921)
  cfblk5/1(emi_1922) -> emi_1853/1, cyemi_990/1
  emi_1925/1 -> cfblk5/Action
  emi_1925/2 -> emi_1923/Action
  emi_1926/1 -> emi_1925/1

== system sampleModel7126_pp_1_1/cfblk283 ==
  cfblk1 : Inport
  cfblk14 : Inport  Port=2
  Action Port : ActionPort  ActionType=then
  cfblk10 : DiscreteTransferFcn
  cfblk11 : DiscreteZeroPole  Poles=[0 0.5]  Gain=1  SampleTime=-1
  cfblk12 : Subsystem  TreatAsAtomicUnit=on
  cfblk13 : Delay  DelayLengthSource=Input port
      settings: InputPortMap=u0,p1
  cfblk3 : simulink/Discrete/Difference  ICPrevInput=0.0  OutMin=[]  OutMax=[]  OutDataTypeStr=double  OutputDataTypeScalingMode=double  OutDataType=fixdt(1, 16)  OutScaling=2^-10  DoSatur=off
  cfblk4 : Subsystem  TreatAsAtomicUnit=on
  cfblk5 : simulink/Discrete/Transfer Fcn Lead or Lag  PoleZ=0.95  ZeroZ=0.75  ICPrevOutput=0.0  ICPrevInput=0.0  DoSatur=off
      settings: SourceProductName=Simulink  SourceProductBaseCode=SL
  cfblk6 : simulink/Discrete/Difference  ICPrevInput=0.0  OutMin=[]  OutMax=[]  OutDataTypeStr=double  OutputDataTypeScalingMode=double  OutDataType=fixdt(1, 16)  OutScaling=2^-10  DoSatur=off
  cfblk7 : Subsystem  TreatAsAtomicUnit=on
  cfblk8 : simulink/Continuous/PID Controller  Controller=PID  TimeDomain=Discrete-time  SampleTime=-1  IntegratorMethod=Forward Euler  FilterMethod=Forward Euler  Form=Parallel  UseFilter=on  ControllerParametersSource=internal  P=1  I=1  D=0  N=100  InitialConditionSource=internal  InitialConditionForIntegrator=0  InitialConditionForFilter=0  ExternalReset=none  LimitOutput=off  UpperSaturationLimit=inf  LowerSaturationLimit=-inf  LinearizeAsGain=off  AntiWindupMode=none  Kb=1  TrackingMode=off  Kt=1  PParamMin=[]  PParamMax=[]  IParamMin=[]  IParamMax=[]  DParamMin=[]  DParamMax=[]  NParamMin=[]  NParamMax=[]  KbParamMin=[]  KbParamMax=[]  KtParamMin=[]  KtParamMax=[]  POutMin=[]  POutMax=[]  IOutMin=[]  IOutMax=[]  DOutMin=[]  DOutMax=[]  NOutMin=[]  NOutMax=[]  KbOutMin=[]  KbOutMax=[]  KtOutMin=[]  KtOutMax=[]  IntegratorOutMin=[]  IntegratorOutMax=[]  FilterOutMin=[]  FilterOutMax=[]  SumOutMin=[]  SumOutMax=[]  SumI1OutMin=[]  SumI1OutMax=[]  SumI2OutMin=[]  SumI2OutMax=[]  SumI3OutMin=[]  SumI3OutMax=[]  SumDOutMin=[]  SumDOutMax=[]  SaturationOutMin=[]  SaturationOutMax=[]  IntegratorContinuousStateAttributes=''  IntegratorStateMustResolveToSignalObject=off  IntegratorRTWStateStorageClass=Auto  FilterContinuousStateAttributes=''  FilterStateMustResolveToSignalObject=off  FilterRTWStateStorageClass=Auto  DifferentiatorICPrevScaledInput=0  DifferentiatorOutMin=[]  DifferentiatorOutMax=[]  FilterDiffOutCoefMin=[]  FilterDiffOutCoefMax=[]  SumDenOutMin=[]  SumDenOutMax=[]  SumNumOutMin=[]  SumNumOutMax=[]  ReciprocalOutMin=[]  ReciprocalOutMax=[]  DivideOutMin=[]  DivideOutMax=[]  TunerSelectOption=Transfer Function Based (PID Tuner App)
  cfblk9 : Subsystem  TreatAsAtomicUnit=on
  cyemi_{1001..1012} (12 alike) : DataTypeConversion  OutDataTypeStr=double
  emi_1012 : Subsystem  TreatAsAtomicUnit=on
  emi_{177,836,1014,1622} (4 alike) : If  IfExpression=Inf <= u1  SampleTime=[1 0]
  emi_{178,837,1015,1623} (4 alike) : DataTypeConversion  OutDataTypeStr=double
  emi_1620 : Subsystem  TreatAsAtomicUnit=on
  emi_175 : Subsystem  TreatAsAtomicUnit=on
  emi_834 : Subsystem  TreatAsAtomicUnit=on
  cfblk2 : Outport
  cfblk15 : Outport  Port=2
  cfblk16 : Outport  Port=3
  cfblk17 : Outport  Port=4
  wires:
  cfblk14/1 -> cfblk2/1, cyemi_1012/1
  cfblk10/1 -> cfblk17/1, cyemi_1005/1, emi_1623/1
  cfblk8/1 -> cyemi_1001/1, cyemi_1002/1
  cyemi_1001/1 -> cfblk10/1
  cyemi_1002/1 -> cfblk11/1
  cfblk13/1 -> cyemi_1003/1
  cyemi_1004/1 -> cfblk13/1
  cfblk3/1 -> cyemi_1004/1
  cyemi_1005/1 -> cfblk13/2
  cyemi_1006/1 -> cfblk3/1
  cfblk11/1 -> cyemi_1006/1, emi_178/1, emi_1015/1
  cfblk5/1 -> cyemi_1007/1
  cyemi_1008/1 -> cfblk5/1
  cfblk6/1 -> cyemi_1008/1
  cyemi_1009/1 -> cfblk6/1
  cfblk1/1 -> cyemi_1010/1
  cyemi_1011/1 -> cfblk8/1
  cyemi_1003/1 -> cfblk12/1(emi_173)
  cfblk12/1(emi_174) -> cyemi_1009/1, emi_837/1
  emi_177/1 -> cfblk12/Action
  emi_177/2 -> emi_175/Action
  emi_178/1 -> emi_177/1
  cyemi_1012/1 -> cfblk9/1(emi_832)
  cfblk9/1(emi_833) -> cfblk16/1
  emi_836/1 -> cfblk9/Action
  emi_836/2 -> emi_834/Action
  emi_837/1 -> emi_836/1
  cyemi_1007/1 -> cfblk4/1(emi_1010)
  cfblk4/1(emi_1011) -> cfblk15/1
  emi_1014/1 -> cfblk4/Action
  emi_1014/2 -> emi_1012/Action
  emi_1015/1 -> emi_1014/1
  cyemi_1010/1 -> cfblk7/1(emi_1618)
  cfblk7/1(emi_1619) -> cyemi_1011/1
  emi_1622/1 -> cfblk7/Action
  emi_1622/2 -> emi_1620/Action
  emi_1623/1 -> emi_1622/1
